simulink model "PV_MEV"  (R2025a)
settings: Solver=VariableStepAuto  StartTime=0.0  StopTime=1  RelTol=1e-3
InitFcn:
  | init_paras
model workspace (MAT data in the model file):
  atk_params = [0 1 0.85 999 0 50 0 0]
  atk_params_vdc = [0 1 0.85 999 0 50 0 0]
values from neighbouring files (symbols this model uses):
  C_PFC = 2600e-6    (= 0.0026)    [init_paras.m]
  ENABLE_HIL = 0    [init_paras.m]
  estimation_src = 1    [init_paras.m]
  Fnom = 50    [init_paras.m]
  Fr_I = Fnom*2    (= 100)    [init_paras.m]
  Ki_V = 80    [init_paras.m]
  Kp_I = 0.06    [init_paras.m]
  Kp_V = 0.25    [init_paras.m]
  Kr_I = 2.5    [init_paras.m]
  L_PFC = 600e-6    (= 0.0006)    [init_paras.m]
  Limit_V = 100    [init_paras.m]
  mm_10cycle_points = mm_points_per_cycle * 10    (= 800)    [init_paras.m]
  mm_fund_freq = 50    [init_paras.m]
  mm_points_per_cycle = 80    [init_paras.m]
  RL_PFC = 20e-3    (= 0.02)    [init_paras.m]
  Ro = 22.22    [init_paras.m]
  Ts_Control = 1/Fc    (= 5e-05)    [init_paras.m]
  Ts_Power = 50e-9    (= 5e-08)    [init_paras.m]
  use_d_predict = 1    [init_paras.m]
  use_harmonic = 1    [init_paras.m]
  use_p_predict = 0    [init_paras.m]
  Vnom_ac = 240    [init_paras.m]
undefined symbols (not defined in the file or in its folder): D1, Delta, DiscIntNeverNeededParam
libraries: spsSeriesRLCBranchLib x17, spsMeanLib x16, spsCurrentMeasurementLib x9, spsFourierLib x8, spsTHDLib x8, spsVoltageMeasurementLib x8, spsDiodeLib x7, MyLibrary x6, instrumentlib x6, pycoexlib x6, simulink x6, spsPWMGeneratorDCDCLib x4
(part 1 of 6)
settings Model: Creator=changhong  LastModifiedBy=changhong
settings DebuggingCC: UnderspecifiedInitializationDetection=Classic  MergeDetectMultiDrivingBlocksExec=none
settings ModelReferenceCC: PropagateSignalLabelsOutOfModel=off

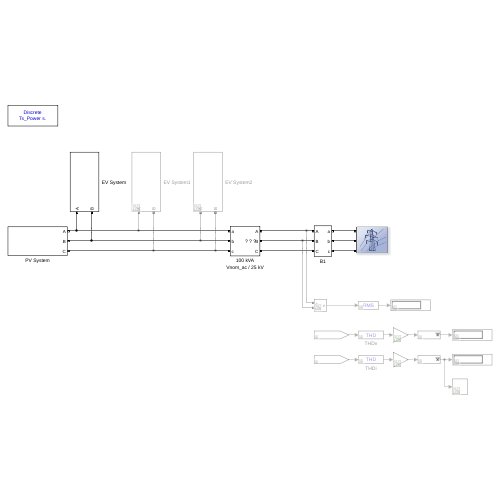
[thumbnail: Simulink's stored preview of the top-level diagram]
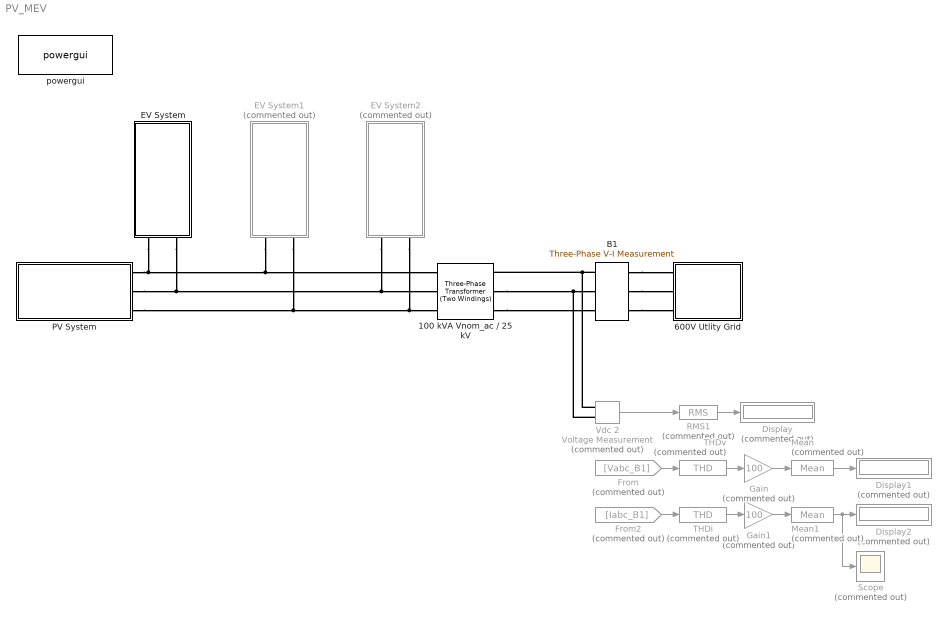
== system PV_MEV ==
  100 kVA Vnom_ac / 25 kV : spsThreePhaseTransformerTwoWindingsLib/Three-Phase Transformer (Two Windings)  Winding1Connection=Y  Winding2Connection=Delta (D1)  CoreType=Three single-phase transformers  SetSaturation=off  Hysteresis=off  DataFile='hysteresis'  SetInitialFlux=off  Measurements=None  UNITS=pu  NominalPower=[100e3 , Fnom ]  Winding1=[ 25e3 , 0.001 , 0.03 ]  Winding2=[ Vnom_ac , 0.001 , 0.03 ]  Rm=500  Lm=500  L0=0.5  Saturation=[ 0,0 ; 0.0024,1.2 ; 1.0,1.52 ]  InitialFluxes=[ 0.8 , -0.8 , 0.7 ]  BreakLoop=off  DiscreteSolver=Trapezoidal iterative  DataType=off  TransfoNumber=0
  600V Utlity Grid : Subsystem
      mask Display: image('$imagefile')
  B1 : spsThreePhaseVIMeasurementLib/Three-Phase V-I Measurement  VoltageMeasurement=phase-to-ground  SetLabelV=on  LabelV=Vabc_B1  Vpu=off  VpuLL=off  CurrentMeasurement=yes  SetLabelI=on  LabelI=Iabc_B1  Ipu=off  Pbase=100e6  Vbase=500e3  OutputType=Magnitude  PhasorSimulation=off  PSBequivalent=0
  Display : Display  Commented=on
  Display1 : Display  Commented=on
  Display2 : Display  Commented=on
  EV System : Subsystem
  EV System1 : Subsystem  Commented=on
  EV System2 : Subsystem  Commented=on
  From : From  Commented=on  GotoTag=Vabc_B1  TagVisibility=global
  From2 : From  Commented=on  GotoTag=Iabc_B1  TagVisibility=global
  Gain : Gain  Commented=on  Gain=100
  Gain1 : Gain  Commented=on  Gain=100
  Mean : spsMeanLib/Mean  Commented=on  Freq=Fnom  Vinit=0  Ts=1/4000
  Mean1 : spsMeanLib/Mean  Commented=on  Freq=Fnom  Vinit=0  Ts=1/4000
  PV System : Subsystem
  RMS1 : spsRMSLib/RMS  Commented=on  TrueRMS=on  Freq=Fnom  RMSInit=0  Ts=0
  Scope : Scope  Commented=on
      settings: ActiveDisplayYMinimum=-25.251011192755687  ActiveDisplayYMaximum=227.25910073480125  DataLoggingVariableName=ScopeData6
  THDi : spsTHDLib/THD  Commented=on  Freq=Fnom  Ts=Ts_Control
  THDv : spsTHDLib/THD  Commented=on  Freq=Fnom  Ts=Ts_Control
  Vdc 2 : spsVoltageMeasurementLib/Voltage Measurement  Tag=PoWeRsYsTeMmEaSuReMeNt  Commented=on  PhasorSimulation=off  OutputType=Magnitude  PSBequivalent=0
  powergui : spspowerguiLib/powergui  Priority=1  SimulationMode=Discrete  SampleTime=Ts_Power  frequency=60  Iterations=50  frequencyindice=0  Pbase=100e6  ErrMax=1e-4  UnitsV=kV  UnitsW=MW  buscounter=0  FunctionMessages=off  echomessages=off  EnableUseOfTLC=off  CurrentSourceSwitches=off  DisableSnubberDevices=off  DisableRonSwitches=off  DisableVfSwitches=off  DisplayEquations=off  AutomaticDiscreteSolvers=off  SolverType=Tustin/Backward Euler (TBE)  Interpol=off  ExternalGateDelay=off  methode=off  Ts=0  x0status=blocks  SPID=off  SwTol=0  HookPort=off  NonlinearTolerance=1e-8  nMaxIteration=10  ContinueOnMaxIteration=off  RestoreLinks=warning  ResistiveCurrentMeasurement=off  Frange=[0:2:500]  Ylog=off  Xlog=on  ShowGrid=off  save=off  variable=ZData  structure=0  ZoomFFT=on  StartTime=0.0  cycles=1  DisplayStyle=1  fundamental=60  FreqAxis=off  MaxFrequency=1000  frequencyindicesteady=1  RmsSteady=1  display=off
  wires:
  Vdc 2/1 -> RMS1/1
  RMS1/1 -> Display/1
  From/1 -> THDv/1
  From2/1 -> THDi/1
  Gain/1 -> Mean/1
  THDv/1 -> Gain/1
  Mean/1 -> Display1/1
  Mean1/1 -> Scope/1, Display2/1
  Gain1/1 -> Mean1/1
  THDi/1 -> Gain1/1
  connections:
  B1/LConn1 -- 100 kVA Vnom_ac / 25 kV/LConn1 -- Vdc 2/LConn1
  100 kVA Vnom_ac / 25 kV/LConn2 -- Vdc 2/LConn2 -- B1/LConn2
  100 kVA Vnom_ac / 25 kV/LConn3 -- B1/LConn3
  B1/RConn1 -- 600V Utlity Grid/LConn1
  B1/RConn2 -- 600V Utlity Grid/LConn2
  B1/RConn3 -- 600V Utlity Grid/LConn3
  PV System/RConn1 -- EV System1/LConn1 -- 100 kVA Vnom_ac / 25 kV/RConn1 -- EV System/LConn1
  PV System/RConn2 -- EV System2/LConn1 -- 100 kVA Vnom_ac / 25 kV/RConn2 -- EV System/LConn2
  PV System/RConn3 -- EV System1/LConn2 -- EV System2/LConn2 -- 100 kVA Vnom_ac / 25 kV/RConn3
